simulink model "read_AS5600_using_arduino_due"  (R2024b)
settings: Solver=FixedStepAuto  StartTime=0.0  StopTime=Inf  RelTol=1e-3  EnableMultiTasking=on
libraries: arduinolib x7, hdlsllib x2
settings Model: ExtModeTrigDuration=2  Creator=leoni  LastModifiedBy=leoni
settings SolverCC: AutoInsertRateTranBlk=on
settings OptimizationCC: EnhancedBackFolding=on  PassReuseOutputArgsAs=Individual arguments  ZeroExternalMemoryAtStartup=off  ZeroInternalMemoryAtStartup=off  MaxStackSize=64  OptimizeBlockOrder=speed  DifferentSizesBufferReuse=on  OptimizationCustomize=off  EfficientTunableParamExpr=on
settings DebuggingCC: ParameterTunabilityLossMsg=error
settings HardwareCC: ProdBitPerPointer=32  ProdBitPerSizeT=32  ProdBitPerPtrDiffT=32  ProdLargestAtomicInteger=Long  ProdLargestAtomicFloat=Double  ProdWordSize=32  ProdHWDeviceType=ARM Compatible->ARM Cortex
settings SFSimCC: MATLABDynamicMemAlloc=off
settings RTWCC: Description=Embedded Coder  SystemTargetFile=ert.tlc  HardwareBoard=Arduino Due  TemplateMakefile=ert_default_tmf  Toolchain=Arduino ARM  BuildConfiguration=Faster Runs
settings CodeAppCC: ForceParamTrailComments=on  IgnoreCustomStorageClasses=off  OperatorAnnotations=on  SimulinkDataObjDesc=on  SFDataObjDesc=on  InsertBlockDesc=on
settings ERTTargetCC: SupportContinuousTime=on  SupportVariableSizeSignals=on  ExtModeTransport=3  ExtModeStaticAlloc=on  ExtModeAutomaticAllocSize=off  ExtModeStaticAllocSize=24576  ExtModeMexFile=ext_xcp  ExtModeIntrfLevel=Level2 - Open  InlinedParameterPlacement=Hierarchical

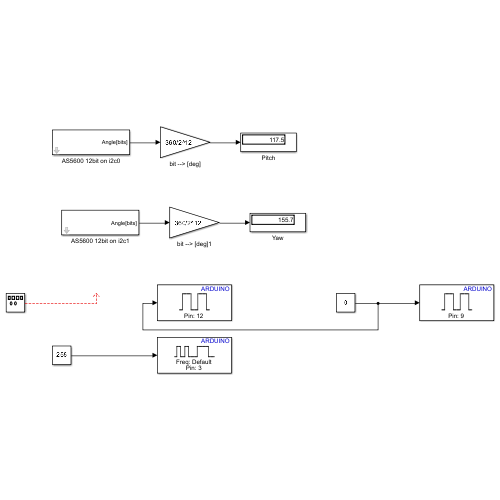
[thumbnail: Simulink's stored preview of the top-level diagram]
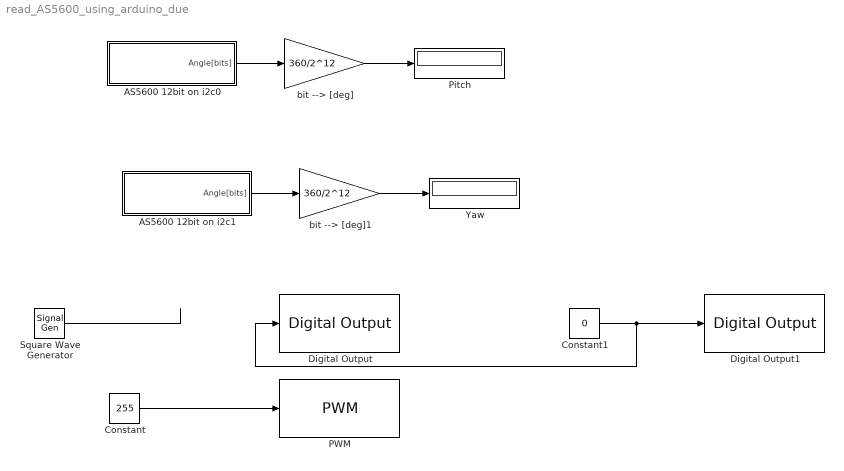
== system read_AS5600_using_arduino_due ==
  AS5600 12bit on i2c0 : Subsystem  mask{deviceAddress=0x36, angleRegAddress=0x0C, ts=0.01}
      mask prompts: deviceAddress "AS 5600 Address"; angleRegAddress "Angle register"; ts "Read Time Step"
  AS5600 12bit on i2c1 : Subsystem  mask{deviceAddress=0x36, angleRegAddress=0x0C, ts=0.01}
      mask prompts: deviceAddress "AS 5600 Address"; angleRegAddress "Angle register"; ts "Read Time Step"
  Constant : Constant  Value=255
  Constant1 : Constant  Value=0
  Digital Output : arduinolib/Digital Output  pinNumber=12  Direction=output  blockPlatform=arduino
      settings: SourceProductName=Common
  Digital Output1 : arduinolib/Digital Output  pinNumber=9  Direction=output  blockPlatform=arduino
      settings: SourceProductName=Common
  PWM : arduinolib/PWM  pinNumber=3  frequencyType=Default  desiredFrequency=490.2  achievableFrequency=490.2
      settings: SourceProductName=Common
  Pitch : Display
  Square Wave Generator : SignalGenerator  WaveForm=square  Frequency=0.1
  Yaw : Display
  bit --> [deg] : Gain  Gain=360/2^12
  bit --> [deg]1 : Gain  Gain=360/2^12
  wires:
  bit --> [deg]/1 -> Pitch/1
  AS5600 12bit on i2c0/1(Angle[bits]) -> bit --> [deg]/1
  bit --> [deg]1/1 -> Yaw/1
  AS5600 12bit on i2c1/1(Angle[bits]) -> bit --> [deg]1/1
  Constant/1 -> PWM/1
  Square Wave Generator/1 -> ?
  Constant1/1 -> Digital Output/1, Digital Output1/1

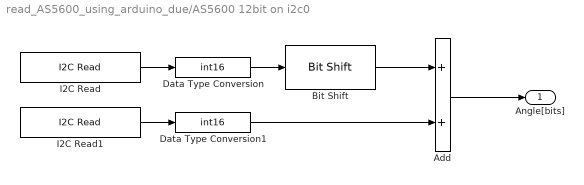
== system read_AS5600_using_arduino_due/AS5600 12bit on i2c0 ==
  Add : Sum
  Bit Shift : hdlsllib/Logic and Bit Operations/Bit Shift  mode=Shift Left Logical  N=8
  Data Type Conversion : DataTypeConversion  OutDataTypeStr=int16  SaturateOnIntegerOverflow=off  RndMeth=Floor
  Data Type Conversion1 : DataTypeConversion  OutDataTypeStr=int16  SaturateOnIntegerOverflow=off  RndMeth=Floor
  I2C Read : arduinolib/I2C Read  I2CModule=0  Mode=Master  SlaveAddress=deviceAddress  SlaveByteOrder=BigEndian  Direction=Receiver  RegisterAddressMode=on  RegisterAddress=angleRegAddress  SlaveDataType=uint8  DataLength=1  NoAck=off  RepeatedStart=off  OutputStatus=off  blockPlatform=ARDUINO  SampleTime=ts
      settings: SourceProductName=Common
  I2C Read1 : arduinolib/I2C Read  I2CModule=0  Mode=Master  SlaveAddress=deviceAddress  SlaveByteOrder=BigEndian  Direction=Receiver  RegisterAddressMode=on  RegisterAddress=angleRegAddress+1  SlaveDataType=uint8  DataLength=1  NoAck=off  RepeatedStart=off  OutputStatus=off  blockPlatform=ARDUINO  SampleTime=ts
      settings: SourceProductName=Common
  Angle[bits] : Outport
  wires:
  Data Type Conversion1/1 -> Add/2
  Bit Shift/1 -> Add/1
  Data Type Conversion/1 -> Bit Shift/1
  I2C Read/1 -> Data Type Conversion/1
  I2C Read1/1 -> Data Type Conversion1/1
  Add/1 -> Angle[bits]/1

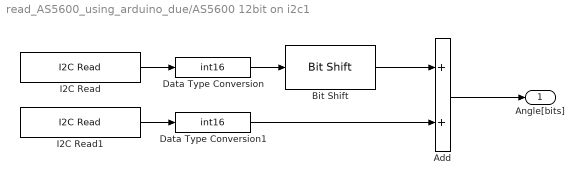
== system read_AS5600_using_arduino_due/AS5600 12bit on i2c1 ==
  Add : Sum
  Bit Shift : hdlsllib/Logic and Bit Operations/Bit Shift  mode=Shift Left Logical  N=8
  Data Type Conversion : DataTypeConversion  OutDataTypeStr=int16  SaturateOnIntegerOverflow=off  RndMeth=Floor
  Data Type Conversion1 : DataTypeConversion  OutDataTypeStr=int16  SaturateOnIntegerOverflow=off  RndMeth=Floor
  I2C Read : arduinolib/I2C Read  I2CModule=1  Mode=Master  SlaveAddress=deviceAddress  SlaveByteOrder=BigEndian  Direction=Receiver  RegisterAddressMode=on  RegisterAddress=angleRegAddress  SlaveDataType=uint8  DataLength=1  NoAck=off  RepeatedStart=off  OutputStatus=off  blockPlatform=ARDUINO  SampleTime=ts
      settings: SourceProductName=Common
  I2C Read1 : arduinolib/I2C Read  I2CModule=1  Mode=Master  SlaveAddress=deviceAddress  SlaveByteOrder=BigEndian  Direction=Receiver  RegisterAddressMode=on  RegisterAddress=angleRegAddress+1  SlaveDataType=uint8  DataLength=1  NoAck=off  RepeatedStart=off  OutputStatus=off  blockPlatform=ARDUINO  SampleTime=ts
      settings: SourceProductName=Common
  Angle[bits] : Outport
  wires:
  Data Type Conversion1/1 -> Add/2
  Bit Shift/1 -> Add/1
  Data Type Conversion/1 -> Bit Shift/1
  I2C Read/1 -> Data Type Conversion/1
  I2C Read1/1 -> Data Type Conversion1/1
  Add/1 -> Angle[bits]/1
